simulink model "Requriment11"  (R2021a)
settings: Solver=FixedStepDiscrete  StartTime=0.0  StopTime=50  FixedStep=1  RelTol=1e-3
libraries: simulink x3
settings Model: Creator=Rahul  LastModifiedBy=Rahul

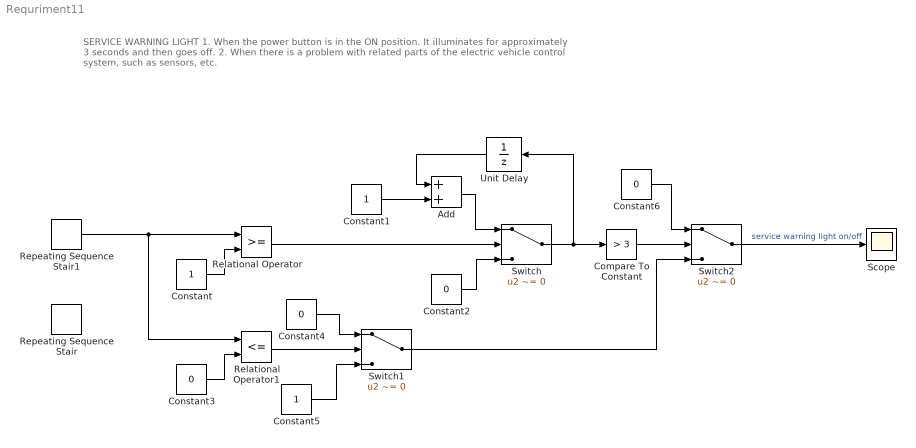
== system Requriment11 ==
  note: SERVICE WARNING LIGHT
      | 1. When the power button is in the ON position.
      | It illuminates for approximately 3 seconds and then goes off.
      | 2. When there is a problem with related parts of the electric vehicle control system, such as sensors, etc.
  Add : Sum
  Compare To Constant : simulink/Logic and Bit Operations/Compare To Constant  relop=>  const=3  OutDataTypeStr=boolean
  Constant : Constant
  Constant1 : Constant
  Constant{2..4,6} (4 alike) : Constant  Value=0
  Constant5 : Constant
  Relational Operator : RelationalOperator  OutDataTypeStr=boolean  RndMeth=Simplest
  Relational Operator1 : RelationalOperator  Operator=<=  OutDataTypeStr=boolean  RndMeth=Simplest
  Repeating Sequence Stair : simulink/Sources/Repeating Sequence Stair  OutValues="[1 1 1 1  0 1 0 1 0]"  tsamp=-1  OutMin=[]  OutMax=[]  OutDataTypeStr=double  OutputDataTypeScalingMode=double  OutDataType=fixdt(0,8)  ConRadixGroup=Best Precision: Vector-wise  OutScaling=2^-12
  Repeating Sequence Stair1 : simulink/Sources/Repeating Sequence Stair  OutValues=[1 1 1 1 0 0 0 1 1 1 1 0 0 0]  tsamp=-1  OutMin=[]  OutMax=[]  OutDataTypeStr=double  OutputDataTypeScalingMode=double  OutDataType=fixdt(0,8)  ConRadixGroup=Best Precision: Vector-wise  OutScaling=2^-12
  Scope : Scope
  Switch : Switch  Criteria=u2 ~= 0
  Switch1 : Switch  Criteria=u2 ~= 0
  Switch2 : Switch  Criteria=u2 ~= 0
  Unit Delay : UnitDelay  SampleTime=-1  HasFrameUpgradeWarning=on
  wires:
  Repeating Sequence Stair1/1 -> Relational Operator1/1, Relational Operator/1
  Constant/1 -> Relational Operator/2
  Constant1/1 -> Add/2
  Unit Delay/1 -> Add/1
  Add/1 -> Switch/1
  Switch/1 -> Unit Delay/1, Compare To Constant/1
  Constant2/1 -> Switch/3
  Compare To Constant/1 -> Switch2/2
  Relational Operator/1 -> Switch/2
  Constant3/1 -> Relational Operator1/2
  Relational Operator1/1 -> Switch1/2
  Constant4/1 -> Switch1/1
  Constant5/1 -> Switch1/3
  Constant6/1 -> Switch2/1
  Switch1/1 -> Switch2/3
  Switch2/1 -> Scope/1  "service warning light on/off"
